simulink model "pla_manuell_parity"  (R2024a)
settings: Solver=ode45  StartTime=0.0  StopTime=inf  RelTol=1e-3  EnableMultiTasking=on
settings Model: Creator=nunkesser  LastModifiedBy=nunkesser
settings SolverCC: AlgebraicLoopSolver=TrustRegion
settings DataIOCC: LimitDataPoints=on  SaveFormat=Array  ReturnWorkspaceOutputs=off
settings OptimizationCC: LifeSpan=inf
settings DebuggingCC: SolverPrmCheckMsg=warning  UnconnectedInputMsg=warning  UnconnectedOutputMsg=warning  UnconnectedLineMsg=warning  SFUnexpectedBacktrackingDiag=warning  SFNoUnconditionalDefaultTransitionDiag=warning  SFExecutionAtInitializationDiag=none  ArithmeticOperatorsInVariantConditions=warning
settings HardwareCC: ProdBitPerPointer=32  ProdBitPerSizeT=32  ProdBitPerPtrDiffT=32  ProdLargestAtomicFloat=None  ProdIntDivRoundTo=Undefined  ProdEndianess=Unspecified  ProdWordSize=32  ProdHWDeviceType=32-bit Generic
settings ModelReferenceCC: PropagateSignalLabelsOutOfModel=off
settings SFSimCC: SimUseLocalCustomCode=off  CustomCodeUndefinedFunction=UseInterfaceOnly
settings RTWCC: RTWUseLocalCustomCode=off  GPUComputeCapability=3.5
settings CodeAppCC: StateflowObjectComments=on
settings GRTTargetCC: TargetLangStandard=C89/C90 (ANSI)
settings ConfigComp: CovMetricSettings=dw  CovSaveCumulativeToWorkspaceVar=on  CovSaveSingleToWorkspaceVar=on  CovExternalEMLEnable=off  CovSFcnEnable=off

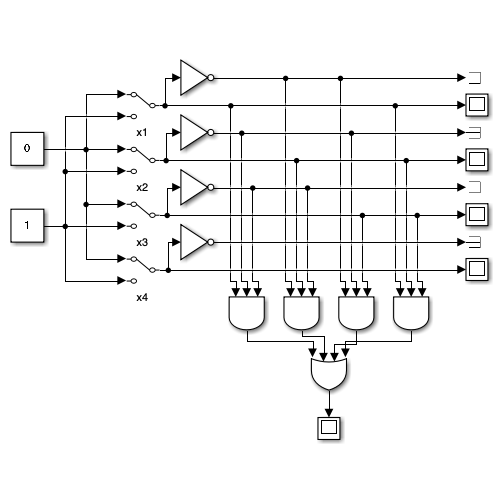
[thumbnail: Simulink's stored preview of the top-level diagram]
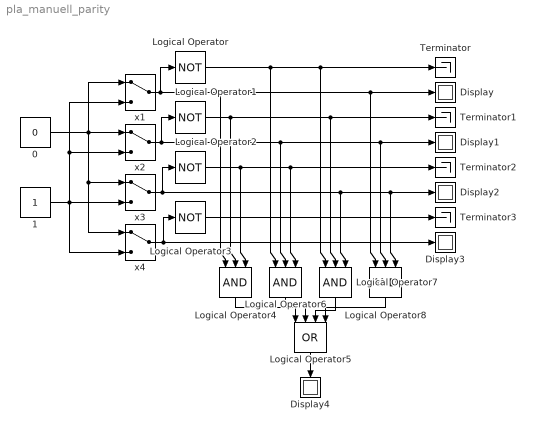
== system pla_manuell_parity ==
  0 : Constant  Value=0  OutDataTypeStr=boolean
  1 : Constant  OutDataTypeStr=boolean
  Display{,1..4} (5 alike) : Display
  Logical Operator{,1..3} (4 alike) : Logic  Operator=NOT  IconShape=distinctive  AllPortsSameDT=off  OutDataTypeStr=boolean
  Logical Operator{4,6..8} (4 alike) : Logic  Inputs=3  IconShape=distinctive  AllPortsSameDT=off  OutDataTypeStr=boolean
  Logical Operator5 : Logic  Operator=OR  Inputs=4  IconShape=distinctive  AllPortsSameDT=off  OutDataTypeStr=boolean
  Terminator{,1..3} (4 alike) : Terminator
  x{1..4} (4 alike) : ManualSwitch
  wires:
  0/1 -> x4/1, x3/1, x2/1, x1/1
  1/1 -> x4/2, x2/2, x1/2, x3/2
  x1/1 -> Logical Operator/1, Logical Operator4/1, Logical Operator8/1, Display/1
  x2/1 -> Logical Operator1/1, Logical Operator6/2, Logical Operator8/2, Display1/1
  x3/1 -> Logical Operator2/1, Logical Operator7/3, Logical Operator8/3, Display2/1
  x4/1 -> Logical Operator3/1, Display3/1
  Logical Operator/1 -> Logical Operator6/1, Logical Operator7/1, Terminator/1
  Logical Operator1/1 -> Logical Operator4/2, Logical Operator7/2, Terminator1/1
  Logical Operator2/1 -> Logical Operator4/3, Logical Operator6/3, Terminator2/1
  Logical Operator3/1 -> Terminator3/1
  Logical Operator5/1 -> Display4/1
  Logical Operator4/1 -> Logical Operator5/1
  Logical Operator6/1 -> Logical Operator5/2
  Logical Operator7/1 -> Logical Operator5/3
  Logical Operator8/1 -> Logical Operator5/4
